simulink model "model"  (R2022b)
settings: Solver=VariableStepAuto  StartTime=0.0  StopTime=40.0  RelTol=1e-3
values from neighbouring files (symbols this model uses):
  J = get_linearization()    [LQG.m]
  Kr = lqr(J.A,J.B,Q,R)    [LQG.m]
undefined symbols (not defined in the file or in its folder): Ke, std_dev_dx, std_dev_dy, std_dev_phi_dot, std_dev_psi, X_start
libraries: simulink x2
settings Model: Creator=alexi  LastModifiedBy=franc

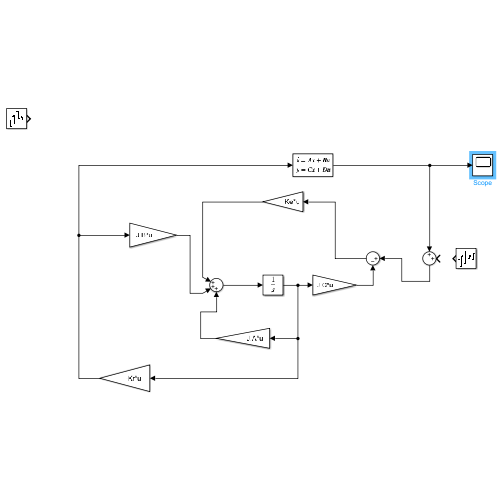
[thumbnail: Simulink's stored preview of the top-level diagram]
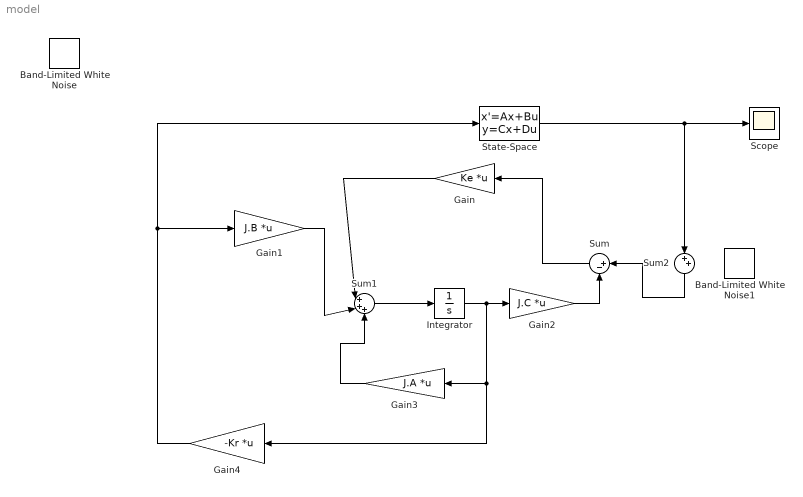
== system model ==
  Band-Limited White Noise : simulink/Sources/Band-Limited White Noise  Cov=[0.1]  Ts=0.1  seed=[23341]
  Band-Limited White Noise1 : simulink/Sources/Band-Limited White Noise  Cov=[std_dev_dx; std_dev_dy; std_dev_phi_dot; std_dev_psi]  Ts=0.1  seed=[23341]
  Gain : Gain  Gain=Ke  Multiplication=Matrix(K*u)
  Gain1 : Gain  Gain=J.B  Multiplication=Matrix(K*u)
  Gain2 : Gain  Gain=J.C  Multiplication=Matrix(K*u)
  Gain3 : Gain  Gain=J.A  Multiplication=Matrix(K*u)
  Gain4 : Gain  Gain=-Kr  Multiplication=Matrix(K*u)
  Integrator : Integrator
  Scope : Scope
  State-Space : StateSpace  A=J.A  B=J.B  C=J.C  D=J.D  InitialCondition=X_start
  Sum : Sum  Inputs=|+-
  Sum1 : Sum  Inputs=|+++
  Sum2 : Sum  Inputs=|++
  wires:
  Gain4/1 -> State-Space/1, Gain1/1
  State-Space/1 -> Scope/1, Sum2/1
  Gain/1 -> Sum1/1
  Gain1/1 -> Sum1/2
  Sum1/1 -> Integrator/1
  Integrator/1 -> Gain4/1, Gain3/1, Gain2/1
  Gain2/1 -> Sum/2
  Gain3/1 -> Sum1/3
  Sum2/1 -> Sum/1
  Sum/1 -> Gain/1
